simulink model "energiebilanz"  (R2013a)
settings: Solver=ode3  StartTime=0.0  StopTime=10.0  RelTol=1e-3
libraries: Thermolib x12
settings Model: Creator=Admin  LastModifiedBy=Admin
settings DataIOCC: ExternalInput=[timet, u]

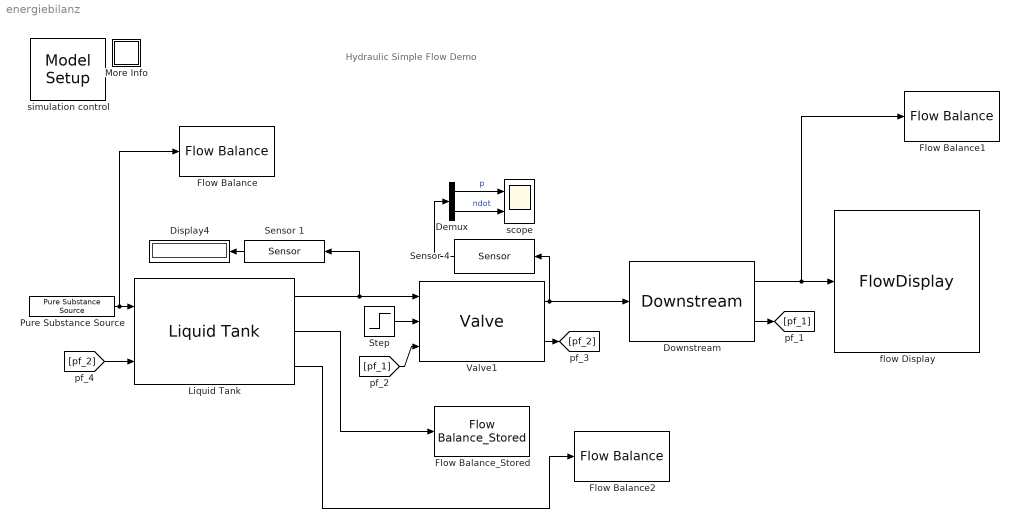
== system energiebilanz ==
  note: Hydraulic Simple Flow Demo
  Demux : Demux  Outputs=2
  Display4 : Display
  Downstream : Thermolib/Components/Hydraulic with Pressure Feedback/Downstream  P=3e5  show_info_port=off  default_order_in_ports={'in'}  default_order_out_ports={'out','PFout','info'}
  Flow Balance : Thermolib/Balance/Flow Balance  asklabel=Use name of parent system  mainlabel='Name here'  direction=in  label='Eintritt'
  Flow Balance1 : Thermolib/Balance/Flow Balance  asklabel=Use name of parent system  mainlabel='Name here'  direction=out  label='Austritt'
  Flow Balance2 : Thermolib/Balance/Flow Balance  asklabel=Use name of parent system  mainlabel='Name here'  direction=out  label='Input flow 1'
  Flow Balance_Stored : Thermolib/Balance/Flow Balance_Stored  asklabel=Use name of parent system  mainlabel=Thermolib/Components/Tanks/Adiabatic Tank  direction=stored  label='tank content'
  Liquid Tank : Thermolib/Components/Tanks/Liquid Tank  Initial_Mass=1e6  T_init=273+25  p_init=5e5  psi_init=[0 1 0 0 0 0 0 0 0]  mdot_out_method=m.out = f(PF)  species_local={'H2O'}  psi_local=1  m_min=10  m_max=400e6  Tank_Model=0  mdot_out_pf_initial=500  mdot_out_pf_max=1000  mdot_out_pf_relaxation=50  default_order_in_ports={'in','PFin','mdot_out'}  default_order_out_ports={'out','state','overflow','PFout','info'}  show_info_port=off  show_PF_port=off
  More Info : Subsystem
      settings: OpenFcn=showdemo(gcs)
      mask Display: disp('?')
  Pure Substance Source : Thermolib/Sources/Pure Substance Source  disp_str=fprintf('H2O Mass flow')  flow_type=Mass flow  switch_flow_type=3  ndot=5 g/s  ndot_in=5  T=298.15 C  T_in=25  p=500000 bar  p_in=5  T_p_x_switch=2  x=1e-005  species_local={'H2O'}  psi_local=1  psi=[0 1 0 0 0 0 0 0 0]
  Sensor 1 : Thermolib/Miscellaneous/Sensor  lst_physical_value=p measured in bar;  mult_fac=1e-05  add_fac=0  selected_signals=3
  Sensor 4 : Thermolib/Miscellaneous/Sensor  lst_physical_value=p measured in Pa;ndot measured in mol/s;  mult_fac=[1 1]  add_fac=[0 0]  selected_signals=[3 1]
  Step : Step  Time=100  Before=0.4  After=0.6  SampleTime=0
  Valve1 : Thermolib/Components/Hydraulic/Valve  valve_type=passive (calculates pressure loss based on Kv-method)  p_downstream_min=0.1e5  P_Loss_1=[0 3 10]  valve_pos_1=[0 0.2 1]  P_Loss_2=[0 3 10]*1e4  valve_pos_2=[0 0.3 1]  Kv_Valve="[16  10 0]*0.1"  valve_pos=[0 0.3 1]  x_local=0  psi_local=1  species_local={'H2O'}  T_initial=300  p_initial=1e5  default_order_in_ports={'in','pos','outlet press.','PFin'}  default_order_out_ports={'out','mdot','dp','PFout','info'}  show_pl_port=off  show_pf_ports=on  show_info_port=off
  flow Display : Thermolib/Sinks/FlowDisplay  bus_type=FlowBus  mdot=off kg/s  m_unit=mg  ndot=on mol/s  n_unit=mmol  temperature=on  T_unit=Kelvin  pressure=on  p_unit=Pa  enthalpy=on  Hdot_unit=W  H_unit=mJ  entropy=on  Sdot_unit=W/K  S_unit=mJ/K  gibbs_energy=on  Gdot_unit=W  G_unit=mJ  heat_capacity=on  Cpdot_unit=W/K  Cp_unit=mJ/K  energy_content=off  U_unit=mW/K  vapor_fraction=off  molar_fraction=off  flag=0.2964
  scope : Scope  NumInputPorts=2
      settings: TimeRange=200  YMin=50000~10  YMax=300000~30
  simulation control : Thermolib/Setup/Model Setup  starttime=0  endtime=100  loadWS=on  loadWSCommand=fc_LoadWorkspace  media_file=ChemicalMediaData.mat  constants_file=Constants.mat  species_reduced={'CH4', 'H2O', 'CO', 'CO2', 'H2', 'N2', 'O2', 'isooctane', 'Methanol'}  load_model_command=load ComponentData.mat  gas_eos_method=1  gas_mixing_rule=0  species_allow_liquid=[1 1 1 1 1 1 1 1 1]  species_allow_vapor=[1 1 1 1 1 1 1 1 1]  last_saved_thermolib_version=5.1.2.5490  liquid_eos_method=1  density_calculation_mode=0
  wires:
  Valve1/1 -> Downstream/1, Sensor 4/1
  Downstream/1 -> Flow Balance1/1, flow Display/1
  Downstream/2 -> [pf_1]
  [pf_1] -> Valve1/3
  Sensor 4/1 -> Demux/1
  Demux/1 -> scope/1  "p"
  Demux/2 -> scope/2  "ndot"
  Step/1 -> Valve1/2
  Valve1/2 -> [pf_2]
  Liquid Tank/1 -> Sensor 1/1, Valve1/1
  Pure Substance Source/1 -> Flow Balance/1, Liquid Tank/1
  Liquid Tank/3 -> Flow Balance2/1
  Sensor 1/1 -> Display4/1
  [pf_2] -> Liquid Tank/2
  Liquid Tank/2 -> Flow Balance_Stored/1

== system energiebilanz/More Info ==
